simulink model "lab2_2"  (R2020a)
settings: Solver=VariableStepAuto  StartTime=0.0  StopTime=10.0  RelTol=1e-3
settings Model: Creator=huang  LastModifiedBy=huang

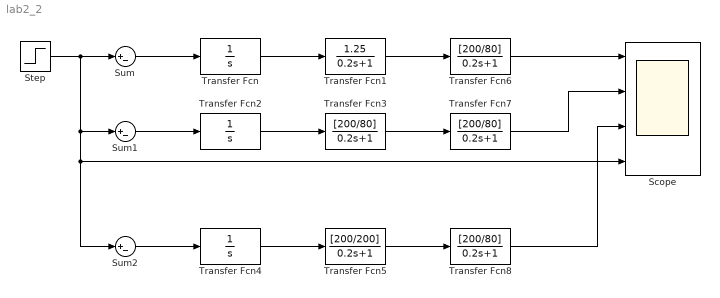
== system lab2_2 ==
  Scope : Scope  NumInputPorts=4
  Step : Step  Time=0  SampleTime=0
  Sum : Sum  Inputs=|+-
  Sum1 : Sum  Inputs=|+-
  Sum2 : Sum  Inputs=|+-
  Transfer Fcn : TransferFcn  Denominator=[1 0]
  Transfer Fcn1 : TransferFcn  Numerator=[1.25]  Denominator=[0.2 1]
  Transfer Fcn2 : TransferFcn  Denominator=[1 0]
  Transfer Fcn{3,6..8} (4 alike) : TransferFcn  Numerator=[200/80]  Denominator=[0.2 1]
  Transfer Fcn4 : TransferFcn  Denominator=[1 0]
  Transfer Fcn5 : TransferFcn  Numerator=[200/200]  Denominator=[0.2 1]
  wires:
  Sum1/1 -> Transfer Fcn2/1
  Transfer Fcn2/1 -> Transfer Fcn3/1
  Transfer Fcn4/1 -> Transfer Fcn5/1
  Sum2/1 -> Transfer Fcn4/1
  Sum/1 -> Transfer Fcn/1
  Transfer Fcn/1 -> Transfer Fcn1/1
  Step/1 -> Sum2/1, Scope/4, Sum1/1, Sum/1
  Transfer Fcn1/1 -> Transfer Fcn6/1
  Transfer Fcn3/1 -> Transfer Fcn7/1
  Transfer Fcn5/1 -> Transfer Fcn8/1
  Transfer Fcn6/1 -> Scope/1
  Transfer Fcn7/1 -> Scope/2
  Transfer Fcn8/1 -> Scope/3
